simulink model "Question_3"  (R2024b)
settings: Solver=FixedStepAuto  StartTime=0.0  StopTime=34  RelTol=1e-3
settings Model: Creator=Sagar  LastModifiedBy=Sagar

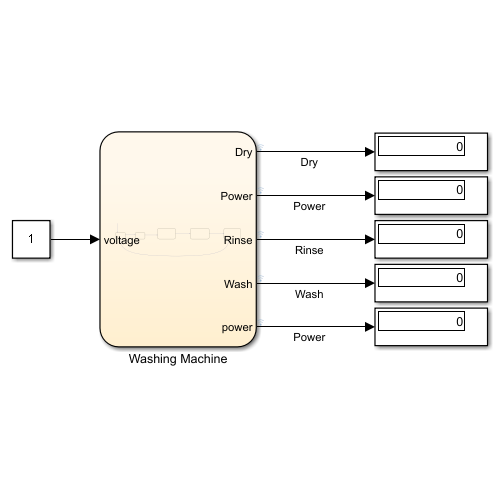
[thumbnail: Simulink's stored preview of the top-level diagram]
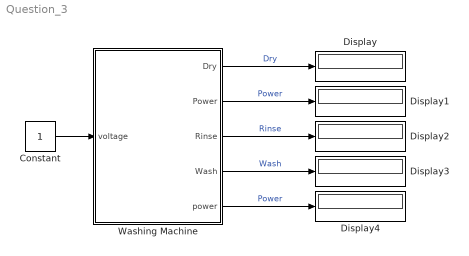
== system Question_3 ==
  Constant : Constant  VectorParams1D=off
  Display{,1..4} (5 alike) : Display
  Washing Machine : Stateflow chart  TreatAsAtomicUnit=on
  wires:
  Constant/1 -> Washing Machine/1(voltage)
  Washing Machine/1(Dry) -> Display/1  "Dry"
  Washing Machine/2(Power) -> Display1/1  "Power"
  Washing Machine/3(Rinse) -> Display2/1  "Rinse"
  Washing Machine/4(Wash) -> Display3/1  "Wash"
  Washing Machine/5(power) -> Display4/1  "Power"

== stateflow chart Question_3/Washing Machine ==
  state Washing
    Wash=1;
  state Rinsing
    entry:
    Rinse=1;
  state Drying
    entry:
    cycle = 1
  state OFF
    power=0;
  state ON
  (default) -> OFF : {cycle=0}
  Washing -> Rinsing : after(20,sec) {Wash=0;Rinse = 1}
  Rinsing -> Drying : after(10,sec){Rinse=0;Dry=1}
  OFF -> ON : [voltage==1&&cycle<1]{power=1}
  ON -> Washing : after(1,sec) {Wash=1}
  Drying -> OFF : after(3,sec)
      | {Power=0;Dry=0}
  data: Dry output; Power output; Rinse output; Wash output; power output; voltage input; cycle local
